simulink library "lib_accessory"  (Simulink 7.9)
settings: Solver=ode45  SolverMode=SingleTasking  StartTime=0.0  StopTime=10.0  RelTol=1e-3
undefined symbols (not defined in the file or in its folder): acc_dcdc_eff, acc_elec_eff, acc_elec_efficiency, acc_elec_pwr, acc_mech_eff, acc_mech_pwr, acc_mech_trq, acc_sindafile, amb_tmp, cyc_mph, ess_on, fc_on, fd_ratio, gb_ratio, load_on, map_spd, max_pwr, pwr_map, tc_gc_to_fc_ratio, time_step, vc_idle_bool, vc_idle_spd, vinf, wh_radius
libraries: lib_accessory x47, lib_cosimulation x29, lib_outputs x11, sub_lib_models x2, simulink3 x2
(part 2 of 3)

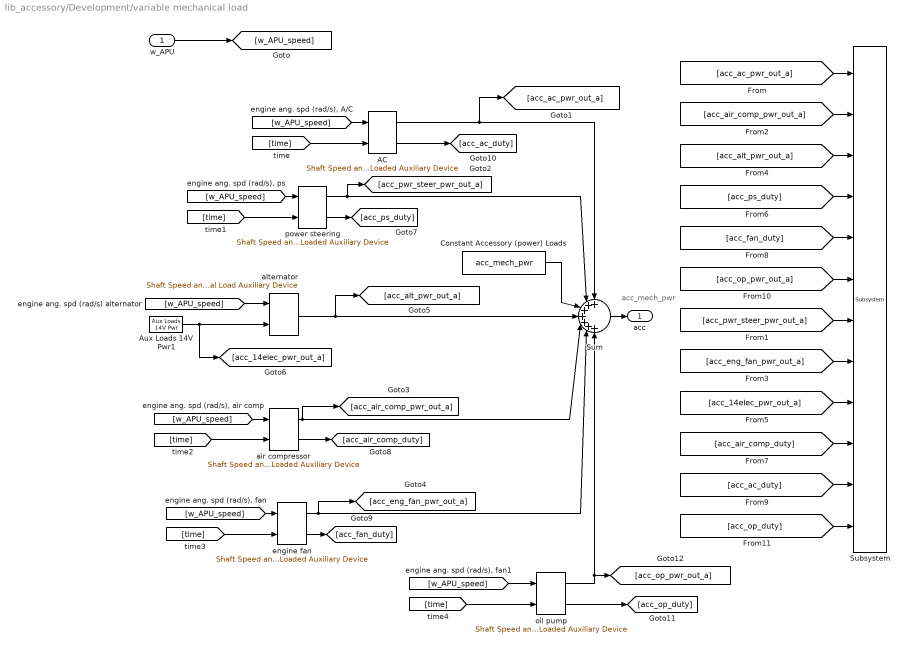
== system lib_accessory/Development/variable mechanical load ==
  note: acc_mech_pwr
  w_APU : Inport
  AC : lib_accessory/SubLibraries/Shaft Speed and Time Loaded Auxiliary Device  acc_duty=acc_ac_dutycycle  pwr_func=acc_ac_pwr_func
  Aux Loads 14V Pwr1 : sub_lib_models/Aux Loads 14V Pwr
      settings: RTWFcnNameOpts=Auto  RTWFileNameOpts=Auto
  Constant Accessory (power) Loads : Constant  Value=acc_mech_pwr
  Subsystem : lib_accessory/SubLibraries/variable accessory load power consumption calculations for conventional mechanical sys. --simulink implementation--/Subsystem
      settings: RTWFcnNameOpts=Auto  RTWFileNameOpts=Auto
  Sum : Sum  Inputs=+++++++  SaturateOnIntegerOverflow=on  InputSameDT=on  OutDataTypeStr=Inherit: Same as first input
  air compressor : lib_accessory/SubLibraries/Shaft Speed and Time Loaded Auxiliary Device  acc_duty=acc_abc_dutycycle  pwr_func=acc_abc_pwr_func
  alternator : lib_accessory/SubLibraries/Shaft Speed and Actual Load Auxiliary Device  conv_eff=acc_acdc_inverter_eff  pwr_func=acc_alt_pwr_func
  engine fan : lib_accessory/SubLibraries/Shaft Speed and Time Loaded Auxiliary Device  acc_duty=acc_ef_dutycycle  pwr_func=acc_ef_pwr_func
  oil pump : lib_accessory/SubLibraries/Shaft Speed and Time Loaded Auxiliary Device  acc_duty=acc_op_dutycycle  pwr_func=acc_op_pwr_func
  power steering : lib_accessory/SubLibraries/Shaft Speed and Time Loaded Auxiliary Device  acc_duty=acc_ps_dutycycle  pwr_func=acc_ps_pwr_func
  acc : Outport
  wires:
  [time] -> AC/2
  [w_APU_speed] -> AC/1
  AC/2 -> [acc_ac_duty]
  AC/1 -> Sum/1, [acc_ac_pwr_out_a]
  Constant Accessory (power) Loads/1 -> Sum/3
  Sum/1 -> acc/1
  [w_APU_speed] -> alternator/1
  air compressor/2 -> [acc_air_comp_duty]
  air compressor/1 -> Sum/5, [acc_air_comp_pwr_out_a]
  [w_APU_speed] -> air compressor/1
  [time] -> air compressor/2
  alternator/1 -> [acc_alt_pwr_out_a], Sum/4
  oil pump/1 -> [acc_op_pwr_out_a], Sum/7
  oil pump/2 -> [acc_op_duty]
  [time] -> oil pump/2
  [w_APU_speed] -> oil pump/1
  engine fan/2 -> [acc_fan_duty]
  [time] -> engine fan/2
  engine fan/1 -> Sum/6, [acc_eng_fan_pwr_out_a]
  [w_APU_speed] -> engine fan/1
  power steering/2 -> [acc_ps_duty]
  [w_APU_speed] -> power steering/1
  [time] -> power steering/2
  power steering/1 -> Sum/2, [acc_pwr_steer_pwr_out_a]
  w_APU/1 -> [w_APU_speed]
  Aux Loads 14V Pwr1/1 -> alternator/2, [acc_14elec_pwr_out_a]
  [acc_ac_pwr_out_a] -> Subsystem/1
  [acc_air_comp_pwr_out_a] -> Subsystem/2
  [acc_alt_pwr_out_a] -> Subsystem/3
  [acc_ps_duty] -> Subsystem/4
  [acc_fan_duty] -> Subsystem/5
  [acc_op_pwr_out_a] -> Subsystem/6
  [acc_pwr_steer_pwr_out_a] -> Subsystem/7
  [acc_eng_fan_pwr_out_a] -> Subsystem/8
  [acc_14elec_pwr_out_a] -> Subsystem/9
  [acc_air_comp_duty] -> Subsystem/10
  [acc_ac_duty] -> Subsystem/11
  [acc_op_duty] -> Subsystem/12

== system lib_accessory/Elec Aux Loads 14V Pwr/BrakeLights ==
  Average Watts : Constant  Value=vinf.AuxLoads.BrakeLights.AverageWatts
  Constant : Constant  Value=0
  Constant1 : Constant
  On : Constant  Value=vinf.AuxLoads.BrakeLights.On
  Product : Product  Inputs=4  SaturateOnIntegerOverflow=on  RndMeth=Zero  InputSameDT=on  OutDataTypeStr=Inherit: Same as first input
  Switch : Switch  SaturateOnIntegerOverflow=on  InputSameDT=on
  Out1 : Outport
  wires:
  Product/1 -> Out1/1
  Constant/1 -> Switch/1
  [F_req] -> Switch/2
  Constant1/1 -> Switch/3
  Average Watts/1 -> Product/4
  [key_on] -> Product/3
  On/1 -> Product/1
  Switch/1 -> Product/2

== system lib_accessory/Elec Aux Loads 14V Pwr/Engine ==
  Average Watts : Constant  Value=vinf.AuxLoads.Engine.AverageWatts
  Memory : Memory
  On : Constant  Value=vinf.AuxLoads.Engine.On
  Product : Product  Inputs=4  SaturateOnIntegerOverflow=on  RndMeth=Zero  InputSameDT=on  OutDataTypeStr=Inherit: Same as first input
  Out1 : Outport
  wires:
  Memory/1 -> Product/2
  [engine_on] -> Memory/1
  [key_on] -> Product/3
  On/1 -> Product/1
  Product/1 -> Out1/1
  Average Watts/1 -> Product/4

== system lib_accessory/Elec Aux Loads 14V Pwr/ExternalLights ==
  Average Watts : Constant  Value=vinf.AuxLoads.ExternalLights.AverageWatts
  On : Constant  Value=vinf.AuxLoads.ExternalLights.On
  Product : Product  Inputs=3  SaturateOnIntegerOverflow=on  RndMeth=Zero  InputSameDT=on  OutDataTypeStr=Inherit: Same as first input
  Subsystem : lib_cosimulation/Subsystem  ModelName='ExternalLights'
  Out1 : Outport
  wires:
  Average Watts/1 -> Product/3
  On/1 -> Product/1
  Subsystem/1 -> Product/2
  Product/1 -> Out1/1

== system lib_accessory/Elec Aux Loads 14V Pwr/FrontHVAC ==
  Average Watts : Constant  Value=vinf.AuxLoads.FrontHVAC.AverageWatts
  On : Constant  Value=vinf.AuxLoads.FrontHVAC.On
  Product : Product  Inputs=3  SaturateOnIntegerOverflow=on  RndMeth=Zero  InputSameDT=on  OutDataTypeStr=Inherit: Same as first input
  Subsystem : lib_cosimulation/Subsystem  ModelName='FrontHVAC'
  Out1 : Outport
  wires:
  Average Watts/1 -> Product/3
  On/1 -> Product/1
  Subsystem/1 -> Product/2
  Product/1 -> Out1/1

== system lib_accessory/Elec Aux Loads 14V Pwr/FrontWipers ==
  Average Watts : Constant  Value=vinf.AuxLoads.FrontWipers.AverageWatts
  On : Constant  Value=vinf.AuxLoads.FrontWipers.On
  Product : Product  Inputs=3  SaturateOnIntegerOverflow=on  RndMeth=Zero  InputSameDT=on  OutDataTypeStr=Inherit: Same as first input
  Subsystem : lib_cosimulation/Subsystem  ModelName='FrontWipers'
  Out1 : Outport
  wires:
  Average Watts/1 -> Product/3
  On/1 -> Product/1
  Subsystem/1 -> Product/2
  Product/1 -> Out1/1

== system lib_accessory/Elec Aux Loads 14V Pwr/HeatedSeats ==
  Average Watts : Constant  Value=vinf.AuxLoads.HeatedSeats.AverageWatts
  Num : Constant  Value=vinf.AuxLoads.HeatedSeats.Num
  On : Constant  Value=vinf.AuxLoads.HeatedSeats.On
  Product : Product  Inputs=4  SaturateOnIntegerOverflow=on  RndMeth=Zero  InputSameDT=on  OutDataTypeStr=Inherit: Same as first input
  Subsystem : lib_cosimulation/Subsystem  ModelName='HeatedSeats'
  Out1 : Outport
  wires:
  Subsystem/1 -> Product/3
  Product/1 -> Out1/1
  Average Watts/1 -> Product/4
  On/1 -> Product/1
  Num/1 -> Product/2

== system lib_accessory/Elec Aux Loads 14V Pwr/Misc ==
  Average Watts : Constant  Value=vinf.AuxLoads.Misc.AverageWatts
  On : Constant  Value=vinf.AuxLoads.Misc.On
  Product : Product  Inputs=3  SaturateOnIntegerOverflow=on  RndMeth=Zero  InputSameDT=on  OutDataTypeStr=Inherit: Same as first input
  Out1 : Outport
  wires:
  Average Watts/1 -> Product/3
  [key_on] -> Product/2
  On/1 -> Product/1
  Product/1 -> Out1/1

== system lib_accessory/Elec Aux Loads 14V Pwr/RadiatorCoolingFan ==
  Average Watts : Constant  Value=vinf.AuxLoads.RadiatorCoolingFan.AverageWatts
  On : Constant  Value=vinf.AuxLoads.RadiatorCoolingFan.On
  Product : Product  Inputs=3  SaturateOnIntegerOverflow=on  RndMeth=Zero  InputSameDT=on  OutDataTypeStr=Inherit: Same as first input
  Subsystem : lib_cosimulation/Subsystem  ModelName='RadiatorCoolingFan'
  Out1 : Outport
  wires:
  Average Watts/1 -> Product/3
  On/1 -> Product/1
  Subsystem/1 -> Product/2
  Product/1 -> Out1/1

== system lib_accessory/Elec Aux Loads 14V Pwr/Radio ==
  Average Watts : Constant  Value=vinf.AuxLoads.Radio.AverageWatts
  Num : Constant  Value=vinf.AuxLoads.Radio.Num
  On : Constant  Value=vinf.AuxLoads.Radio.On
  Product : Product  Inputs=4  SaturateOnIntegerOverflow=on  RndMeth=Zero  InputSameDT=on  OutDataTypeStr=Inherit: Same as first input
  Subsystem : lib_cosimulation/Subsystem  ModelName='Radio'
  Out1 : Outport
  wires:
  Subsystem/1 -> Product/3
  Average Watts/1 -> Product/4
  On/1 -> Product/1
  Num/1 -> Product/2
  Product/1 -> Out1/1

== system lib_accessory/Elec Aux Loads 14V Pwr/RearDefrost ==
  Average Watts : Constant  Value=vinf.AuxLoads.RearDefrost.AverageWatts
  On : Constant  Value=vinf.AuxLoads.RearDefrost.On
  Product : Product  Inputs=3  SaturateOnIntegerOverflow=on  RndMeth=Zero  InputSameDT=on  OutDataTypeStr=Inherit: Same as first input
  Subsystem : lib_cosimulation/Subsystem  ModelName='RearDefrost'
  Out1 : Outport
  wires:
  Subsystem/1 -> Product/2
  Average Watts/1 -> Product/3
  On/1 -> Product/1
  Product/1 -> Out1/1

== system lib_accessory/Elec Aux Loads 14V Pwr/RearHVAC ==
  Average Watts : Constant  Value=vinf.AuxLoads.RearHVAC.AverageWatts
  On : Constant  Value=vinf.AuxLoads.RearHVAC.On
  Product : Product  Inputs=3  SaturateOnIntegerOverflow=on  RndMeth=Zero  InputSameDT=on  OutDataTypeStr=Inherit: Same as first input
  Subsystem : lib_cosimulation/Subsystem  ModelName='RearHVAC'
  Out1 : Outport
  wires:
  Average Watts/1 -> Product/3
  On/1 -> Product/1
  Subsystem/1 -> Product/2
  Product/1 -> Out1/1

== system lib_accessory/Elec Aux Loads 14V Pwr/RearWipers ==
  Average Watts : Constant  Value=vinf.AuxLoads.RearWipers.AverageWatts
  On : Constant  Value=vinf.AuxLoads.RearWipers.On
  Product : Product  Inputs=3  SaturateOnIntegerOverflow=on  RndMeth=Zero  InputSameDT=on  OutDataTypeStr=Inherit: Same as first input
  Subsystem : lib_cosimulation/Subsystem  ModelName='RearWipers'
  Out1 : Outport
  wires:
  Average Watts/1 -> Product/3
  On/1 -> Product/1
  Subsystem/1 -> Product/2
  Product/1 -> Out1/1

== system lib_accessory/Elec Aux Loads 14V Pwr/Starter ==
  Product1 : Product  SaturateOnIntegerOverflow=on  RndMeth=Zero  InputSameDT=on  OutDataTypeStr=Inherit: Same as first input
  Starter : lib_cosimulation/14V Load Control/Starter
      settings: RTWFcnNameOpts=Auto  RTWFileNameOpts=Auto
  starter_load (power) : Constant  Value=vinf.AuxLoads.Starter.AverageWatts
  Out1 : Outport
  wires:
  Starter/1 -> Product1/1
  starter_load (power)/1 -> Product1/2
  Product1/1 -> Out1/1

== system lib_accessory/Elec Aux Loads 14V Pwr/TurnSignals ==
  Average Watts : Constant  Value=vinf.AuxLoads.TurnSignals.AverageWatts
  On : Constant  Value=vinf.AuxLoads.TurnSignals.On
  Product : Product  Inputs=3  SaturateOnIntegerOverflow=on  RndMeth=Zero  InputSameDT=on  OutDataTypeStr=Inherit: Same as first input
  Subsystem : lib_cosimulation/Subsystem  ModelName='TurnSignals'
  Out1 : Outport
  wires:
  Average Watts/1 -> Product/3
  On/1 -> Product/1
  Subsystem/1 -> Product/2
  Product/1 -> Out1/1

== system lib_accessory/Elec Aux Loads HiV Pwr/CurrentLoad1 ==
  Average Watts : Constant  Value=vinf.AuxLoads.CurrentLoad1.AverageWatts
  On : Constant  Value=vinf.AuxLoads.CurrentLoad1.On
  Product : Product  Inputs=3  SaturateOnIntegerOverflow=on  RndMeth=Zero  InputSameDT=on  OutDataTypeStr=Inherit: Same as first input
  Subsystem : lib_cosimulation/Subsystem  ModelName='CurrentLoad1'
  Out1 : Outport
  wires:
  Product/1 -> Out1/1
  Subsystem/1 -> Product/2
  On/1 -> Product/1
  Average Watts/1 -> Product/3

== system lib_accessory/Elec Aux Loads HiV Pwr/PowerLoad1 ==
  Average Watts : Constant  Value=vinf.AuxLoads.PowerLoad1.AverageWatts
  On : Constant  Value=vinf.AuxLoads.PowerLoad1.On
  Product : Product  Inputs=3  SaturateOnIntegerOverflow=on  RndMeth=Zero  InputSameDT=on  OutDataTypeStr=Inherit: Same as first input
  Subsystem : lib_cosimulation/Subsystem  ModelName='PowerLoad1'
  Out1 : Outport
  wires:
  Product/1 -> Out1/1
  On/1 -> Product/1
  Average Watts/1 -> Product/3
  Subsystem/1 -> Product/2

== system lib_accessory/Elec Aux Loads HiV Pwr/PowerLoad2 ==
  Average Watts : Constant  Value=vinf.AuxLoads.PowerLoad2.AverageWatts
  On : Constant  Value=vinf.AuxLoads.PowerLoad2.On
  Product : Product  Inputs=3  SaturateOnIntegerOverflow=on  RndMeth=Zero  InputSameDT=on  OutDataTypeStr=Inherit: Same as first input
  Subsystem : lib_cosimulation/Subsystem  ModelName='PowerLoad2'
  Out1 : Outport
  wires:
  Subsystem/1 -> Product/2
  Average Watts/1 -> Product/3
  On/1 -> Product/1
  Product/1 -> Out1/1

== system lib_accessory/Elec Aux Loads HiV Pwr/PowerLoad3 ==
  Average Watts : Constant  Value=vinf.AuxLoads.PowerLoad3.AverageWatts
  On : Constant  Value=vinf.AuxLoads.PowerLoad3.On
  Product : Product  Inputs=3  SaturateOnIntegerOverflow=on  RndMeth=Zero  InputSameDT=on  OutDataTypeStr=Inherit: Same as first input
  Subsystem : lib_cosimulation/Subsystem  ModelName='PowerLoad3'
  Out1 : Outport
  wires:
  Product/1 -> Out1/1
  On/1 -> Product/1
  Average Watts/1 -> Product/3
  Subsystem/1 -> Product/2

== system lib_accessory/Elec Aux Loads HiV Pwr/SpeedLoad1 ==
  On : Constant  Value=vinf.AuxLoads.SpeedLoad1.On
  Product : Product  Inputs=3  SaturateOnIntegerOverflow=on  RndMeth=Zero  InputSameDT=on  OutDataTypeStr=Inherit: Same as first input
  Subsystem : lib_cosimulation/Subsystem  ModelName='SpeedLoad1'
  "rad/s -> rpm1" : Gain  Gain=60/(2*pi)  SaturateOnIntegerOverflow=on  OutDataTypeStr=Inherit: Same as input  ParamDataTypeStr=Inherit: Same as input
  speed (rpm) vs load (watts) : Lookup  InputValues=[vinf.AuxLoads.SpeedLoad1.Data(1,1),vinf.AuxLoads.SpeedLoad1.Data(2,1)]  Table=[vinf.AuxLoads.SpeedLoad1.Data(1,2),vinf.AuxLoads.SpeedLoad1.Data(2,2)]  SaturateOnIntegerOverflow=on
  Out1 : Outport
  wires:
  Product/1 -> Out1/1
  Subsystem/1 -> Product/2
  On/1 -> Product/1
  speed (rpm) vs load (watts)/1 -> Product/3
  [w_APU_speed] -> "rad/s -> rpm1"/1
  "rad/s -> rpm1"/1 -> speed (rpm) vs load (watts)/1

== system lib_accessory/Elec Aux Loads HiV Pwr/Starter ==
  Product1 : Product  SaturateOnIntegerOverflow=on  RndMeth=Zero  InputSameDT=on  OutDataTypeStr=Inherit: Same as first input
  Starter : Subsystem
  starter_load (power) : Constant  Value=vinf.AuxLoads.Starter.AverageWatts
  Out1 : Outport
  wires:
  Product1/1 -> Out1/1
  starter_load (power)/1 -> Product1/2
  Starter/1(Starter_OnOff_Control) -> Product1/1

== system lib_accessory/Electrical Accessory Loads v2 <acc>/Accessory SDO ==
  data bus : Inport
  Demux : Demux  Outputs=3
  To Workspace : ToWorkspace  VariableName=acc_elec_pwr_r  SampleTime=-1
  To Workspace3 : ToWorkspace  VariableName=acc_elec_pwr_a  SampleTime=-1
  To Workspace4 : ToWorkspace  VariableName=acc_elec_pwr_est  SampleTime=-1
  electrical power logging : lib_accessory/SubLibraries/electrical power logging  eff=acc_mech_eff
  wires:
  data bus/1 -> Demux/1
  Demux/1 -> To Workspace/1
  Demux/2 -> To Workspace3/1, electrical power logging/1
  Demux/3 -> To Workspace4/1

== system lib_accessory/Electrical Accessory Loads v2 <acc>/Block NOTES ==
  note: In terms of an interface, the model assumes electrical power generated from
      | a powersource (or powersources)
      |
      | This model takes in requested driveline electrical power output requests and
      | augments power to account for electrically driven accessories.
      |
      | The power passed along down to the driveline is only power to move the
      | vehicle.
  note: This is the electrical auxiliary loads model.

== system lib_accessory/Electrical Accessory Loads v2 <acc>/backward model ==
  note: Pwr, W, powersource out
  note: P, W, for driveline
  note: Power Electrical
      | Accessory
      | (W)
  pwr_in : Inport
  on/off : Inport  Port=2
  Constant : Constant  Value=load_on
  Product : Product  Inputs=***  SaturateOnIntegerOverflow=on  RndMeth=Zero  InputSameDT=on  OutDataTypeStr=Inherit: Same as first input
  Sum : Sum  Inputs=|++  SaturateOnIntegerOverflow=on  InputSameDT=on  OutDataTypeStr=Inherit: Same as first input
  electrical accessories (W) : Subsystem  BlockChoice=Electrical Accessories: Time Variable
      settings: AttributesFormatString=%<BlockChoice>  TemplateBlock=lib_accessory/electrical accessories (W)  MemberBlocks=Electrical Accessories: Constant,Electrical Accessories: Time Variable
      mask Display: image(imread('bdi_acc_elec.bmp'))
  elec_out : Outport
  elec_acc_out : Outport  Port=2
  wires:
  Sum/1 -> elec_out/1
  pwr_in/1 -> Sum/1
  electrical accessories (W)/1(P_elec_acc) -> Product/1
  on/off/1 -> Product/2
  Constant/1 -> Product/3
  Product/1 -> elec_acc_out/1, Sum/2

== system lib_accessory/Electrical Accessory Loads v2 <acc>/forward model ==
  note: Power to driveline
  note: Power Available
  note: electric
      | accessory
      | power (W)
  note: This calculation assumes that the power provider is never so power limited as to
      | not be able to provide at least the value of acc_pwr_in.
  note: ASSUMPTIONS
  pwr_in : Inport
  acc_pwr_in : Inport  Port=2
  Sum : Sum  Inputs=|+-  SaturateOnIntegerOverflow=on  InputSameDT=on  OutDataTypeStr=Inherit: Same as first input
  pwr_out : Outport
  acc_pwr_out : Outport  Port=2
  wires:
  Sum/1 -> pwr_out/1
  pwr_in/1 -> Sum/1
  acc_pwr_in/1 -> Sum/2, acc_pwr_out/1

== system lib_accessory/Mechanical Accessory Loads v2 <acc>/Accessory SDO ==
  data bus : Inport
  Demux : Demux  Outputs=6
  To Workspace : ToWorkspace  VariableName=acc_mech_trq_r  SampleTime=-1
  To Workspace1 : ToWorkspace  VariableName=acc_mech_pwr_a  SampleTime=-1
  To Workspace2 : ToWorkspace  VariableName=acc_mech_trq_est  SampleTime=-1
  To Workspace3 : ToWorkspace  VariableName=acc_mech_pwr_r  SampleTime=-1
  To Workspace4 : ToWorkspace  VariableName=acc_mech_trq_a  SampleTime=-1
  To Workspace5 : ToWorkspace  VariableName=acc_mech_pwr_est  SampleTime=-1
  mechanical power logging : lib_accessory/SubLibraries/mechanical power logging  eff=acc_mech_eff
  wires:
  data bus/1 -> Demux/1
  Demux/4 -> mechanical power logging/1, To Workspace1/1
  Demux/1 -> To Workspace/1
  Demux/2 -> To Workspace3/1
  Demux/3 -> To Workspace4/1
  Demux/5 -> To Workspace2/1
  Demux/6 -> To Workspace5/1

== system lib_accessory/Mechanical Accessory Loads v2 <acc>/Block NOTES ==
  note: This is the mechanical auxiliary loads model.
  note: In terms of an interface, the model assumes belt-driven mechanical loads
      | that run off of a prime mover shaft (e.g., engine shaft)
      |
      | This model takes in requested driveline torque and speed requests and
      | augments torque due to belt driven accessories.
      |
      | The torque passed along down to the driveline is only torque to move the
      | vehicle.
  note: A third input is given for accessory load speed. This is done so that
      | the accessory block can use fc_spd_est which is an estimated vehicle speed
      | (equal to fc_spd_out under normal circumstances).
      | Using fc_spd_est provides total compatibility with ADVISOR v3.2
  note: In this model, only one speed is used to predict accessory
      | loading. The forward model is "dummied" out.

== system lib_accessory/Mechanical Accessory Loads v2 <acc>/backward model ==
  note: w_apu, rad/s
  note: T, Nm, accessory
  note: T, Nm, driveline
  note: T, Nm, shaft out
  note: Power, W, input to accessory
  trq_in : Inport
  spd_in : Inport  Port=2
  acc on/off : Inport  Port=3
  Product : Product  Inputs=**  SaturateOnIntegerOverflow=on  RndMeth=Zero  InputSameDT=on  OutDataTypeStr=Inherit: Same as first input
  Product1 : Product  Inputs=**  SaturateOnIntegerOverflow=on  RndMeth=Zero  InputSameDT=on  OutDataTypeStr=Inherit: Same as first input
  Sum : Sum  Inputs=|++  SaturateOnIntegerOverflow=on  InputSameDT=on  OutDataTypeStr=Inherit: Same as first input
  acc_mech_var_loads : ToWorkspace  VariableName=acc_mech_var_load  SampleTime=-1  SaveFormat=Structure
  mechanical accessories (Nm) : Subsystem  BlockChoice=Mechanical Accessories: Speed Dependant and Variable Electrical
      settings: AttributesFormatString=%<BlockChoice>  TemplateBlock=lib_accessory/mechanical accessories (Nm)  MemberBlocks=Mechanical Accessories: Const Mech Var Elect,Mechanical Accessories: Constant Mechanical & Electrical,Mechanical Accessories: Speed Dependant and Variable Electrical,Saber Dual Voltage Cosim,Saber Single Voltage Cosim,SindaTransAC
      mask Display: image(imread('bdi_acc_pic_cs.bmp'))
  trq_out : Outport
  acc_mech_trq_r : Outport  Port=2
  acc_mech_pwr_r : Outport  Port=3
  wires:
  spd_in/1 -> mechanical accessories (Nm)/1(w_APU)
  trq_in/1 -> Sum/1
  Sum/1 -> trq_out/1
  Product/1 -> acc_mech_trq_r/1, Sum/2
  mechanical accessories (Nm)/1(T_acc) -> Product/2
  Product1/1 -> acc_mech_pwr_r/1
  mechanical accessories (Nm)/2(P_mech_acc) -> Product1/1
  acc on/off/1 -> [acc_on]
  [acc_on] -> Product/1
  [acc_on] -> Product1/2
  mechanical accessories (Nm)/3(probes) -> acc_mech_var_loads/1

== system lib_accessory/Mechanical Accessory Loads v2 <acc>/forward model ==
  note: acc speed, rad/s
  note: T, Nm, accessory
  note: driveline and
      | acc torque, Nm
  note: T, Nm, shaft out
  note: Power, W, input to accessory
  note: This simplistic model may not correctly account for accessory torque and/or power
      | when the upstream torque provider is torque or speed limited
  note: NOTES
  note: acc torque, Nm
  trq_in : Inport
  spd_in : Inport  Port=2
  acc_trq_req : Inport  Port=3
  Product1 : Product  Inputs=**  SaturateOnIntegerOverflow=on  RndMeth=Zero  InputSameDT=on  OutDataTypeStr=Inherit: Same as first input
  Sum : Sum  Inputs=|+-  SaturateOnIntegerOverflow=on  InputSameDT=on  OutDataTypeStr=Inherit: Same as first input
  trq_out : Outport
  acc_mech_trq_a : Outport  Port=2
  acc_mech_pwr_a : Outport  Port=3
  wires:
  spd_in/1 -> [acc_spd]
  Sum/1 -> trq_out/1
  Product1/1 -> acc_mech_pwr_a/1
  [acc_trq_r] -> acc_mech_trq_a/1, Sum/2, Product1/1
  [acc_spd] -> Product1/2
  trq_in/1 -> [pm_trq_a]
  acc_trq_req/1 -> [acc_trq_r]
  [pm_trq_a] -> Sum/1

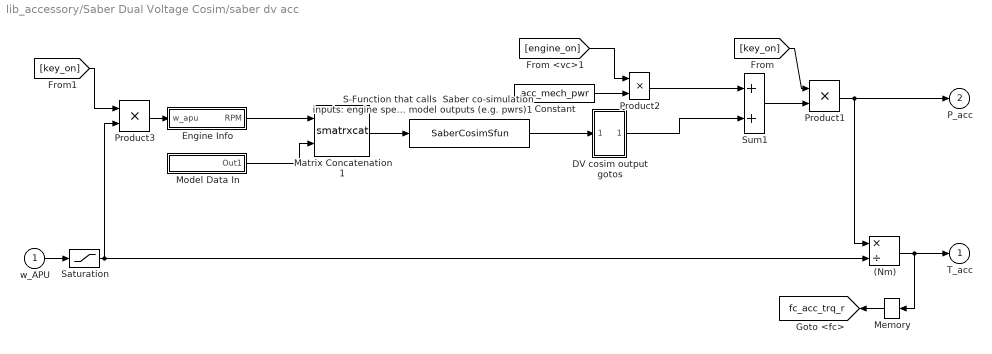
== system lib_accessory/Saber Dual Voltage Cosim/saber dv acc ==
  w_APU : Inport
  (Nm) : Product  Inputs=*/  SaturateOnIntegerOverflow=on  RndMeth=Zero  InputSameDT=on  OutDataTypeStr=Inherit: Same as first input
  Constant : Constant  Value=acc_mech_pwr
  DV cosim output gotos : Subsystem
  Engine Info : Subsystem
  Matrix Concatenation1 : S-Function  FunctionName=smatrxcat  Parameters=numInports,catMethod  EnableBusSupport=off  mask(Matrix Concatenation){numInports=2, catMethod=Horizontal}
      mask prompts: numInports "Number of inputs:"; catMethod "Concatenation method:"
      mask help: Perform horizontal or vertical concatenation. 1-D vector input signals are treated as column vectors, i.e., [Mx1] matrices. The output is always a matrix.
      mask init:
      | xy = matrxcatmask('icon');
      mask StyleString: edit,popup(Horizontal|Vertical)
      mask Display:
      | plot(xy.x,xy.y);
      | text(0.15,0.86,xy.label);
  Memory : Memory
  Model Data In : Subsystem
      mask Display: disp('14V/42V acc')
  Product1 : Product  SaturateOnIntegerOverflow=on  RndMeth=Zero  InputSameDT=on  OutDataTypeStr=Inherit: Same as first input
  Product2 : Product  SaturateOnIntegerOverflow=on  RndMeth=Zero  InputSameDT=on  OutDataTypeStr=Inherit: Same as first input
  Product3 : Product  SaturateOnIntegerOverflow=on  RndMeth=Zero  InputSameDT=on  OutDataTypeStr=Inherit: Same as first input
  S-Function that calls  Saber co-simulation inputs: engine speed (rad/s) load parameters outputs: accessory power model outputs (e.g. pwrs)1 : S-Function  FunctionName=SaberCosimSfun  Parameters=vinf.tmppath,time_step,'SaberCosimIO_DV'  EnableBusSupport=off
  Saturation : Saturate  UpperLimit=inf  LowerLimit=0
  Sum1 : Sum  SaturateOnIntegerOverflow=on  InputSameDT=on  OutDataTypeStr=Inherit: Same as first input
  T_acc : Outport  InitialOutput=0
  P_acc : Outport  Port=2  InitialOutput=0
  tag scope: fc_acc_trq_r=global
  wires:
  Product3/1 -> Engine Info/1(w_apu)
  [key_on] -> Product3/1
  DV cosim output gotos/1(Out1) -> Sum1/2
  Product1/1 -> (Nm)/1, P_acc/1
  [key_on] -> Product1/1
  Sum1/1 -> Product1/2
  Product2/1 -> Sum1/1
  [engine_on] -> Product2/1
  Constant/1 -> Product2/2
  (Nm)/1 -> T_acc/1, Memory/1
  Memory/1 -> [fc_acc_trq_r]
  w_APU/1 -> Saturation/1
  Saturation/1 -> Product3/2, (Nm)/2
  S-Function that calls  Saber co-simulation inputs: engine speed (rad/s) load parameters outputs: accessory power model outputs (e.g. pwrs)1/1 -> DV cosim output gotos/1(In1)
  Matrix Concatenation1/1 -> S-Function that calls  Saber co-simulation inputs: engine speed (rad/s) load parameters outputs: accessory power model outputs (e.g. pwrs)1/1
  Engine Info/1(RPM) -> Matrix Concatenation1/1
  Model Data In/1(Out1) -> Matrix Concatenation1/2

== system lib_accessory/Saber Single Voltage Cosim/saber sv acc ==
  w_APU : Inport
  (Nm) : Product  Inputs=*/  SaturateOnIntegerOverflow=on  RndMeth=Zero  InputSameDT=on  OutDataTypeStr=Inherit: Same as first input
  Constant : Constant  Value=acc_mech_pwr
  Engine Info : Subsystem
  Matrix Concatenation1 : S-Function  FunctionName=smatrxcat  Parameters=numInports,catMethod  EnableBusSupport=off  mask(Matrix Concatenation){numInports=2, catMethod=Horizontal}
      mask prompts: numInports "Number of inputs:"; catMethod "Concatenation method:"
      mask help: Perform horizontal or vertical concatenation. 1-D vector input signals are treated as column vectors, i.e., [Mx1] matrices. The output is always a matrix.
      mask init:
      | xy = matrxcatmask('icon');
      mask StyleString: edit,popup(Horizontal|Vertical)
      mask Display:
      | plot(xy.x,xy.y);
      | text(0.15,0.86,xy.label);
  Memory : Memory
  Product1 : Product  SaturateOnIntegerOverflow=on  RndMeth=Zero  InputSameDT=on  OutDataTypeStr=Inherit: Same as first input
  Product2 : Product  SaturateOnIntegerOverflow=on  RndMeth=Zero  InputSameDT=on  OutDataTypeStr=Inherit: Same as first input
  Product3 : Product  SaturateOnIntegerOverflow=on  RndMeth=Zero  InputSameDT=on  OutDataTypeStr=Inherit: Same as first input
  S-Function that calls  Saber co-simulation inputs: engine speed (rad/s) load parameters outputs: accessory power model outputs (e.g. pwrs) : S-Function  FunctionName=SaberCosimSfun  Parameters=vinf.tmppath,time_step,'SaberCosimIO_SV'  EnableBusSupport=off
  SV Model Data In : Subsystem
      mask Display: disp('14V acc')
  SV cosim output gotos : Subsystem
  Saturation : Saturate  UpperLimit=inf  LowerLimit=0
  Sum1 : Sum  SaturateOnIntegerOverflow=on  InputSameDT=on  OutDataTypeStr=Inherit: Same as first input
  T_acc : Outport  InitialOutput=0
  P_acc : Outport  Port=2  InitialOutput=0
  tag scope: fc_acc_trq_r=global
  wires:
  Product3/1 -> Engine Info/1(w_apu)
  [key_on] -> Product3/1
  SV cosim output gotos/1(Out1) -> Sum1/2
  SV Model Data In/1(Out1) -> Matrix Concatenation1/2
  Engine Info/1(RPM) -> Matrix Concatenation1/1
  Matrix Concatenation1/1 -> S-Function that calls  Saber co-simulation inputs: engine speed (rad/s) load parameters outputs: accessory power model outputs (e.g. pwrs)/1
  S-Function that calls  Saber co-simulation inputs: engine speed (rad/s) load parameters outputs: accessory power model outputs (e.g. pwrs)/1 -> SV cosim output gotos/1(In1)
  Saturation/1 -> Product3/2, (Nm)/2
  w_APU/1 -> Saturation/1
  Memory/1 -> [fc_acc_trq_r]
  (Nm)/1 -> Memory/1, T_acc/1
  Constant/1 -> Product2/2
  [engine_on] -> Product2/1
  Product2/1 -> Sum1/1
  Sum1/1 -> Product1/2
  [key_on] -> Product1/1
  Product1/1 -> P_acc/1, (Nm)/1

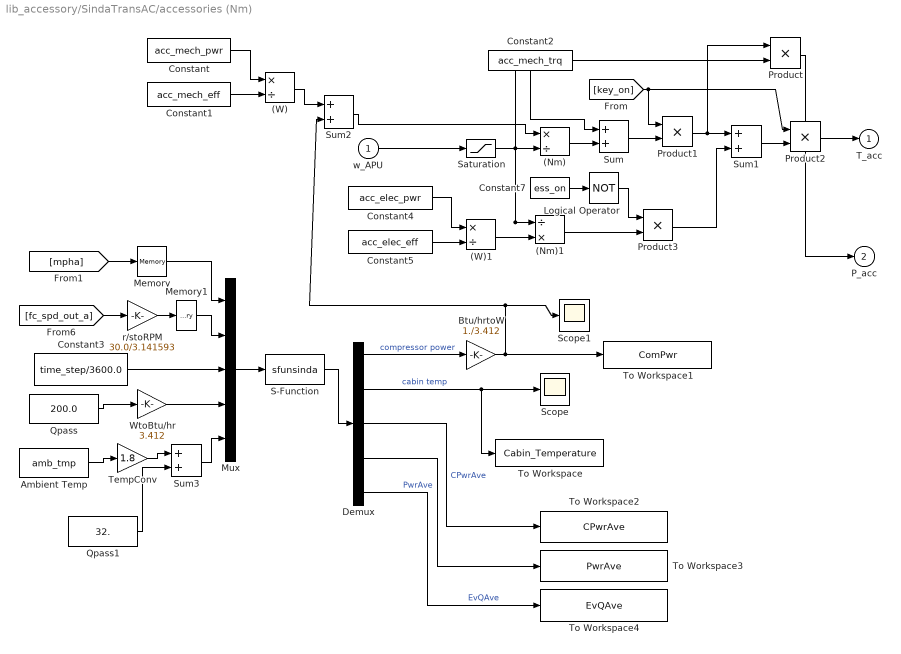
== system lib_accessory/SindaTransAC/accessories (Nm) ==
  w_APU : Inport
  (Nm) : Product  Inputs=*/  SaturateOnIntegerOverflow=on  RndMeth=Zero  InputSameDT=on  OutDataTypeStr=Inherit: Same as first input
  (Nm)1 : Product  Inputs=/*  SaturateOnIntegerOverflow=on  RndMeth=Zero  InputSameDT=on  OutDataTypeStr=Inherit: Same as first input
  (W) : Product  Inputs=*/  SaturateOnIntegerOverflow=on  RndMeth=Zero  InputSameDT=on  OutDataTypeStr=Inherit: Same as first input
  (W)1 : Product  Inputs=*/  SaturateOnIntegerOverflow=on  RndMeth=Zero  InputSameDT=on  OutDataTypeStr=Inherit: Same as first input
  Ambient Temp : Constant  Value=amb_tmp
  Btu/hrtoW : Gain  Gain=1./3.412  SaturateOnIntegerOverflow=on  OutDataTypeStr=Inherit: Same as input  ParamDataTypeStr=Inherit: Same as input
  Constant : Constant  Value=acc_mech_pwr
  Constant1 : Constant  Value=acc_mech_eff
  Constant2 : Constant  Value=acc_mech_trq
  Constant3 : Constant  Value=time_step/3600.0
  Constant4 : Constant  Value=acc_elec_pwr
  Constant5 : Constant  Value=acc_elec_eff
  Constant7 : Constant  Value=ess_on
  Demux : Demux  Outputs=5
  Logical Operator : Logic  Operator=NOT
  Memory : Memory  X0=45.0
  Memory1 : Memory  X0=600.
  Mux : Mux  Inputs=5
  Product{,1..3} (4 alike) : Product  SaturateOnIntegerOverflow=on  RndMeth=Zero  InputSameDT=on  OutDataTypeStr=Inherit: Same as first input
  Qpass : Constant  Value=200.0
  Qpass1 : Constant  Value=32.
  S-Function : S-Function  FunctionName=sfunsinda  Parameters=sindafile  EnableBusSupport=off
  Saturation : Saturate  UpperLimit=inf  LowerLimit=vc_idle_spd+eps
  Scope : Scope
      settings: YMin=130  YMax=170
  Scope1 : Scope
  Sum{,1..3} (4 alike) : Sum  SaturateOnIntegerOverflow=on  InputSameDT=on  OutDataTypeStr=Inherit: Same as first input
  TempConv : Gain  Gain=1.8  SaturateOnIntegerOverflow=on  OutDataTypeStr=Inherit: Same as input  ParamDataTypeStr=Inherit: Same as input
  To Workspace : ToWorkspace  VariableName=Cabin_Temperature  SampleTime=-1
  To Workspace1 : ToWorkspace  VariableName=ComPwr  SampleTime=-1
  To Workspace2 : ToWorkspace  VariableName=CPwrAve  SampleTime=-1
  To Workspace3 : ToWorkspace  VariableName=PwrAve  SampleTime=-1
  To Workspace4 : ToWorkspace  VariableName=EvQAve  SampleTime=-1
  WtoBtu/hr : Gain  Gain=3.412  SaturateOnIntegerOverflow=on  OutDataTypeStr=Inherit: Same as input  ParamDataTypeStr=Inherit: Same as input
  r/stoRPM : Gain  Gain=30.0/3.141593  SaturateOnIntegerOverflow=on  OutDataTypeStr=Inherit: Same as input  ParamDataTypeStr=Inherit: Same as input
  T_acc : Outport  InitialOutput=0
  P_acc : Outport  Port=2  InitialOutput=0
  wires:
  Mux/1 -> S-Function/1
  S-Function/1 -> Demux/1
  [fc_spd_out_a] -> r/stoRPM/1
  Qpass/1 -> WtoBtu/hr/1
  WtoBtu/hr/1 -> Mux/4
  Product1/1 -> Product/1, Sum1/1
  Sum1/1 -> Product2/2
  Logical Operator/1 -> Product3/1
  Product3/1 -> Sum1/2
  Product/1 -> P_acc/1
  (Nm)1/1 -> Product3/2
  Constant7/1 -> Logical Operator/1
  (W)1/1 -> (Nm)1/2
  Constant4/1 -> (W)1/1
  Constant5/1 -> (W)1/2
  Product2/1 -> T_acc/1
  [key_on] -> Product2/1, Product1/1
  Sum/1 -> Product1/2
  (Nm)/1 -> Sum/2
  Saturation/1 -> Product/2, (Nm)1/1, (Nm)/2
  w_APU/1 -> Saturation/1
  Constant2/1 -> Sum/1
  (W)/1 -> Sum2/1
  Sum2/1 -> (Nm)/1
  Constant/1 -> (W)/1
  Constant1/1 -> (W)/2
  Demux/2 -> To Workspace/1, Scope/1  "cabin temp"
  Ambient Temp/1 -> TempConv/1
  TempConv/1 -> Sum3/1
  Qpass1/1 -> Sum3/2
  Sum3/1 -> Mux/5
  Demux/1 -> Btu/hrtoW/1  "compressor power"
  [mpha] -> Memory/1
  Memory/1 -> Mux/1
  r/stoRPM/1 -> Memory1/1
  Memory1/1 -> Mux/2
  Constant3/1 -> Mux/3
  Btu/hrtoW/1 -> Sum2/2, Scope1/1, To Workspace1/1
  Demux/3 -> To Workspace2/1  "CPwrAve"
  Demux/4 -> To Workspace3/1  "PwrAve"
  Demux/5 -> To Workspace4/1  "EvQAve"

== system lib_accessory/SubLibraries/Shaft Speed and Actual Load Auxiliary Device ==
  angular  speed of engine  shaft (rad/s) : Inport
  load on device (W) : Inport  Port=2
  Gain : Gain  Gain=1/conv_eff  SaturateOnIntegerOverflow=on  OutDataTypeStr=Inherit: Same as input  ParamDataTypeStr=Inherit: Same as input
  Mux : Mux  Inputs=2
  device power requirements : MATLABFcn  MATLABFcn=feval(pwr_func, u(1), u(2))  OutputDimensions=1  OutputSignalType=real
  powr required by device (W) : Outport
  wires:
  angular  speed of engine  shaft (rad/s)/1 -> Mux/1
  Gain/1 -> Mux/2
  load on device (W)/1 -> Gain/1
  device power requirements/1 -> powr required by device (W)/1
  Mux/1 -> device power requirements/1

== system lib_accessory/SubLibraries/Shaft Speed and Actual Load Auxiliary Device--lookuptable ==
  angular  speed of engine  shaft (rad/s) : Inport
  load on device (W) : Inport  Port=2
  Constant : Constant  Value=0.0
  Constant1 : Constant  Value=eps
  Gain : Gain  Gain=1/conv_eff  SaturateOnIntegerOverflow=on  OutDataTypeStr=Inherit: Same as input  ParamDataTypeStr=Inherit: Same as input
  Look-Up Table : Lookup  InputValues=map_spd  Table=max_pwr  SaturateOnIntegerOverflow=on
  Look-Up Table (2-D) : simulink3/Functions & Tables/Look-Up Table (2-D)  x=map_spd  y=map_load  t=pwr_map
  Product : Product  Inputs=*/  SaturateOnIntegerOverflow=on  RndMeth=Zero  InputSameDT=on  OutDataTypeStr=Inherit: Same as first input
  Relational Operator : RelationalOperator  Operator=~=  InputSameDT=on
  Saturation : Saturate  UpperLimit=1.0  LowerLimit=0.0
  Saturation1 : Saturate  UpperLimit=maxSpd  LowerLimit=minSpd
  Switch : Switch  Threshold=0.5  SaturateOnIntegerOverflow=on  InputSameDT=on
  powr required by device (W) : Outport
  wires:
  load on device (W)/1 -> Gain/1
  Look-Up Table (2-D)/1 -> powr required by device (W)/1
  angular  speed of engine  shaft (rad/s)/1 -> Saturation1/1
  [spd] -> Look-Up Table (2-D)/1
  Saturation1/1 -> [spd]
  Gain/1 -> Product/1
  [spd] -> Look-Up Table/1
  Product/1 -> Saturation/1
  Saturation/1 -> Look-Up Table (2-D)/2
  Look-Up Table/1 -> Relational Operator/1, Switch/1
  Constant/1 -> Relational Operator/2
  Relational Operator/1 -> Switch/2
  Constant1/1 -> Switch/3
  Switch/1 -> Product/2

== system lib_accessory/SubLibraries/Shaft Speed and Time Loaded Auxiliary Device ==
  angular  speed of engine  shaft (rad/s) : Inport
  elapsed time since start of simulation (s) : Inport  Port=2
  Mux : Mux  Inputs=2
  Sat : Saturate  UpperLimit=1.0  LowerLimit=0.0
  device duty  schedule by time : Subsystem  mask(Repeating table){t=acc_duty(:,1), y=acc_duty(:,2)}
      mask prompts: t "Input values:"; y "Output values:"
      mask help:
      | Repeating table.
      | Enter values of input and output for first cycle.
      mask init:
      | period = max(@1);
      mask Help: Repeats cycle given in table. Input values should be monotonically increasing.
  device power requirements : MATLABFcn  MATLABFcn=feval(pwr_func, u(1), u(2))  OutputDimensions=1  OutputSignalType=real
  powr required by device (W) : Outport
  "duty cycle (1=\"on full power\" & 0=\"off\")" : Outport  Port=2
  wires:
  Mux/1 -> device power requirements/1
  angular  speed of engine  shaft (rad/s)/1 -> Mux/1
  device power requirements/1 -> powr required by device (W)/1
  elapsed time since start of simulation (s)/1 -> device duty  schedule by time/1(distance travelled (m))
  device duty  schedule by time/1(out_1) -> Sat/1
  Sat/1 -> Mux/2, "duty cycle (1=\"on full power\" & 0=\"off\")"/1

== system lib_accessory/SubLibraries/Shaft Speed and Time Loaded Auxiliary Device--lookuptable ==
  angular  speed of engine  shaft (rad/s) : Inport
  elapsed time since start of simulation (s) : Inport  Port=2
  Look-Up Table (2-D) : Lookup2D  RowIndex=map_spd  ColumnIndex=map_load  Table=pwr_map  SaturateOnIntegerOverflow=on  InputSameDT=on
  Sat : Saturate  UpperLimit=1.0  LowerLimit=0.0
  Sat1 : Saturate  UpperLimit=maxSpd  LowerLimit=minSpd
  device duty  schedule by time : Subsystem  mask(Repeating table){t=acc_duty(:,1), y=acc_duty(:,2)}
      mask prompts: t "Input values:"; y "Output values:"
      mask help:
      | Repeating table.
      | Enter values of input and output for first cycle.
      mask init:
      | period = max(t);
      mask Help: Repeats cycle given in table. Input values should be monotonically increasing.
  powr required by device (W) : Outport
  "duty cycle (1=\"on full power\" & 0=\"off\")" : Outport  Port=2
  wires:
  Look-Up Table (2-D)/1 -> powr required by device (W)/1
  elapsed time since start of simulation (s)/1 -> device duty  schedule by time/1(distance travelled (m))
  device duty  schedule by time/1(out_1) -> Sat/1
  Sat/1 -> "duty cycle (1=\"on full power\" & 0=\"off\")"/1, Look-Up Table (2-D)/2
  angular  speed of engine  shaft (rad/s)/1 -> Sat1/1
  Sat1/1 -> Look-Up Table (2-D)/1

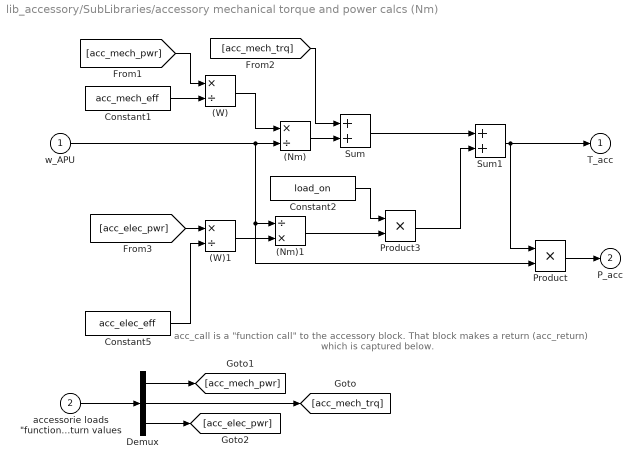
== system lib_accessory/SubLibraries/accessory mechanical torque and power calcs (Nm) ==
  note: acc_call is a "function call" to the
      | accessory block. That block makes
      | a return (acc_return) which is captured below.
  w_APU : Inport
  "accessorie loads \"function\" return values" : Inport  Port=2
  (Nm) : Product  Inputs=*/  SaturateOnIntegerOverflow=on  RndMeth=Zero  InputSameDT=on  OutDataTypeStr=Inherit: Same as first input
  (Nm)1 : Product  Inputs=/*  SaturateOnIntegerOverflow=on  RndMeth=Zero  InputSameDT=on  OutDataTypeStr=Inherit: Same as first input
  (W) : Product  Inputs=*/  SaturateOnIntegerOverflow=on  RndMeth=Zero  InputSameDT=on  OutDataTypeStr=Inherit: Same as first input
  (W)1 : Product  Inputs=*/  SaturateOnIntegerOverflow=on  RndMeth=Zero  InputSameDT=on  OutDataTypeStr=Inherit: Same as first input
  Constant1 : Constant  Value=acc_mech_eff
  Constant2 : Constant  Value=load_on
  Constant5 : Constant  Value=acc_elec_eff
  Demux : Demux  Outputs=3
  Product : Product  SaturateOnIntegerOverflow=on  RndMeth=Zero  InputSameDT=on  OutDataTypeStr=Inherit: Same as first input
  Product3 : Product  SaturateOnIntegerOverflow=on  RndMeth=Zero  InputSameDT=on  OutDataTypeStr=Inherit: Same as first input
  Sum : Sum  SaturateOnIntegerOverflow=on  InputSameDT=on  OutDataTypeStr=Inherit: Same as first input
  Sum1 : Sum  SaturateOnIntegerOverflow=on  InputSameDT=on  OutDataTypeStr=Inherit: Same as first input
  T_acc : Outport  InitialOutput=0
  P_acc : Outport  Port=2  InitialOutput=0
  wires:
  "accessorie loads \"function\" return values"/1 -> Demux/1
  Demux/3 -> [acc_elec_pwr]
  Demux/1 -> [acc_mech_pwr]
  Demux/2 -> [acc_mech_trq]
  Product/1 -> P_acc/1
  (W)/1 -> (Nm)/1
  Constant1/1 -> (W)/2
  [acc_mech_pwr] -> (W)/1
  (Nm)/1 -> Sum/2
  Sum/1 -> Sum1/1
  Sum1/1 -> Product/1, T_acc/1
  Constant5/1 -> (W)1/2
  (W)1/1 -> (Nm)1/2
  (Nm)1/1 -> Product3/2
  Product3/1 -> Sum1/2
  Constant2/1 -> Product3/1
  [acc_mech_trq] -> Sum/1
  w_APU/1 -> (Nm)1/1, Product/2, (Nm)/2
  [acc_elec_pwr] -> (W)1/1

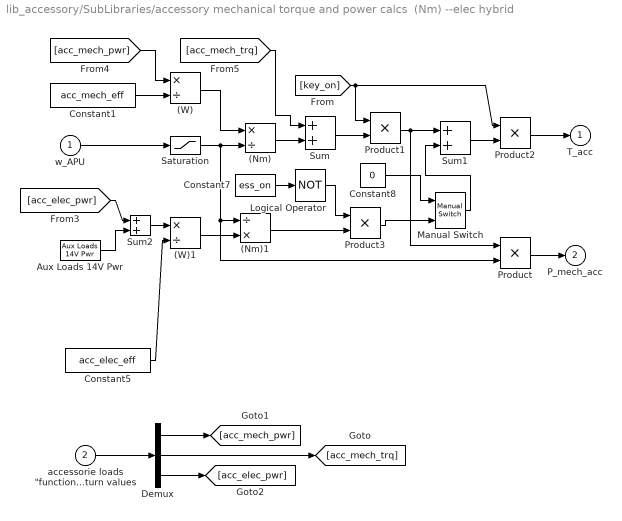
== system lib_accessory/SubLibraries/accessory mechanical torque and power calcs  (Nm) --elec hybrid ==
  w_APU : Inport
  "accessorie loads \"function\" return values" : Inport  Port=2
  (Nm) : Product  Inputs=*/  SaturateOnIntegerOverflow=on  RndMeth=Zero  InputSameDT=on  OutDataTypeStr=Inherit: Same as first input
  (Nm)1 : Product  Inputs=/*  SaturateOnIntegerOverflow=on  RndMeth=Zero  InputSameDT=on  OutDataTypeStr=Inherit: Same as first input
  (W) : Product  Inputs=*/  SaturateOnIntegerOverflow=on  RndMeth=Zero  InputSameDT=on  OutDataTypeStr=Inherit: Same as first input
  (W)1 : Product  Inputs=*/  SaturateOnIntegerOverflow=on  RndMeth=Zero  InputSameDT=on  OutDataTypeStr=Inherit: Same as first input
  Aux Loads 14V Pwr : sub_lib_models/Aux Loads 14V Pwr
      settings: RTWFcnNameOpts=Auto  RTWFileNameOpts=Auto
  Constant1 : Constant  Value=acc_mech_eff
  Constant5 : Constant  Value=acc_elec_eff
  Constant7 : Constant  Value=ess_on
  Constant8 : Constant  Value=0
  Demux : Demux  Outputs=3
  Logical Operator : Logic  Operator=NOT
  Manual Switch : simulink3/Nonlinear/Manual Switch  sw=1  action=0
  Product{,1..3} (4 alike) : Product  SaturateOnIntegerOverflow=on  RndMeth=Zero  InputSameDT=on  OutDataTypeStr=Inherit: Same as first input
  Saturation : Saturate  UpperLimit=inf  LowerLimit=vc_idle_spd+eps
  Sum : Sum  SaturateOnIntegerOverflow=on  InputSameDT=on  OutDataTypeStr=Inherit: Same as first input
  Sum1 : Sum  SaturateOnIntegerOverflow=on  InputSameDT=on  OutDataTypeStr=Inherit: Same as first input
  Sum2 : Sum  SaturateOnIntegerOverflow=on  InputSameDT=on  OutDataTypeStr=Inherit: Same as first input
  T_acc : Outport  InitialOutput=0
  P_mech_acc : Outport  Port=2  InitialOutput=0
  wires:
  Logical Operator/1 -> Product3/1
  (Nm)1/1 -> Product3/2
  Constant7/1 -> Logical Operator/1
  (W)1/1 -> (Nm)1/2
  Constant5/1 -> (W)1/2
  Product2/1 -> T_acc/1
  [key_on] -> Product2/1, Product1/1
  Sum1/1 -> Product2/2
  Sum/1 -> Product1/2
  (Nm)/1 -> Sum/2
  Saturation/1 -> (Nm)/2, Product/2, (Nm)1/1
  w_APU/1 -> Saturation/1
  [acc_mech_pwr] -> (W)/1
  Constant1/1 -> (W)/2
  (W)/1 -> (Nm)/1
  [acc_mech_trq] -> Sum/1
  Product/1 -> P_mech_acc/1
  Product1/1 -> Product/1, Sum1/1
  Product3/1 -> Manual Switch/2
  Manual Switch/1 -> Sum1/2
  Constant8/1 -> Manual Switch/1
  Sum2/1 -> (W)1/1
  [acc_elec_pwr] -> Sum2/1
  Aux Loads 14V Pwr/1 -> Sum2/2
  "accessorie loads \"function\" return values"/1 -> Demux/1
  Demux/3 -> [acc_elec_pwr]
  Demux/1 -> [acc_mech_pwr]
  Demux/2 -> [acc_mech_trq]

== system lib_accessory/SubLibraries/data logging probes dummy ==
  In1 : Inport
  Terminator : Terminator
  wires:
  In1/1 -> Terminator/1

== system lib_accessory/SubLibraries/data logging probes for conventional mechanical loads ==
  In1 : Inport
  Demux : Demux  Outputs=12
  To Workspace : ToWorkspace  VariableName=acc_ac_pwr_out_a  SampleTime=-1
  To Workspace1 : ToWorkspace  VariableName=acc_pwr_steer_pwr_out_a  SampleTime=-1
  To Workspace10 : ToWorkspace  VariableName=acc_op_pwr_out_a  SampleTime=-1
  To Workspace11 : ToWorkspace  VariableName=acc_op_duty  SampleTime=-1
  To Workspace2 : ToWorkspace  VariableName=acc_air_comp_pwr_out_a  SampleTime=-1
  To Workspace3 : ToWorkspace  VariableName=acc_eng_fan_pwr_out_a  SampleTime=-1
  To Workspace4 : ToWorkspace  VariableName=acc_alt_pwr_out_a  SampleTime=-1
  To Workspace5 : ToWorkspace  VariableName=acc_14elec_pwr_out_a  SampleTime=-1
  To Workspace6 : ToWorkspace  VariableName=acc_ps_duty  SampleTime=-1
  To Workspace7 : ToWorkspace  VariableName=acc_air_comp_duty  SampleTime=-1
  To Workspace8 : ToWorkspace  VariableName=acc_fan_duty  SampleTime=-1
  To Workspace9 : ToWorkspace  VariableName=acc_ac_duty  SampleTime=-1
  wires:
  Demux/12 -> To Workspace11/1
  Demux/11 -> To Workspace10/1
  Demux/10 -> To Workspace9/1
  Demux/9 -> To Workspace8/1
  Demux/8 -> To Workspace7/1
  Demux/7 -> To Workspace6/1
  Demux/6 -> To Workspace5/1
  Demux/5 -> To Workspace4/1
  Demux/4 -> To Workspace3/1
  Demux/3 -> To Workspace2/1
  Demux/2 -> To Workspace1/1
  Demux/1 -> To Workspace/1
  In1/1 -> Demux/1

== system lib_accessory/SubLibraries/data probes ==
  In1 : Inport
  data logging probes for conventional mechanical loads : lib_accessory/SubLibraries/data logging probes for conventional mechanical loads
      settings: RTWFcnNameOpts=Auto  RTWFileNameOpts=Auto
  wires:
  In1/1 -> data logging probes for conventional mechanical loads/1

== system lib_accessory/SubLibraries/electrical power logging ==
  In1 : Inport
  Gain : Gain  Gain=acc_elec_eff  SaturateOnIntegerOverflow=on  OutDataTypeStr=Inherit: Same as input  ParamDataTypeStr=Inherit: Same as input
  To Workspace6 : ToWorkspace  VariableName=acc_elec_pwr_in_a  SampleTime=-1
  To Workspace8 : ToWorkspace  VariableName=acc_elec_pwr_out_a  SampleTime=-1
  wires:
  In1/1 -> To Workspace6/1, Gain/1
  Gain/1 -> To Workspace8/1

== system lib_accessory/SubLibraries/mechanical power logging ==
  In1 : Inport
  Gain : Gain  Gain=acc_mech_eff  SaturateOnIntegerOverflow=on  OutDataTypeStr=Inherit: Same as input  ParamDataTypeStr=Inherit: Same as input
  To Workspace6 : ToWorkspace  VariableName=acc_mech_pwr_in_a  SampleTime=-1
  To Workspace8 : ToWorkspace  VariableName=acc_mech_pwr_out_a  SampleTime=-1
  wires:
  In1/1 -> To Workspace6/1, Gain/1
  Gain/1 -> To Workspace8/1

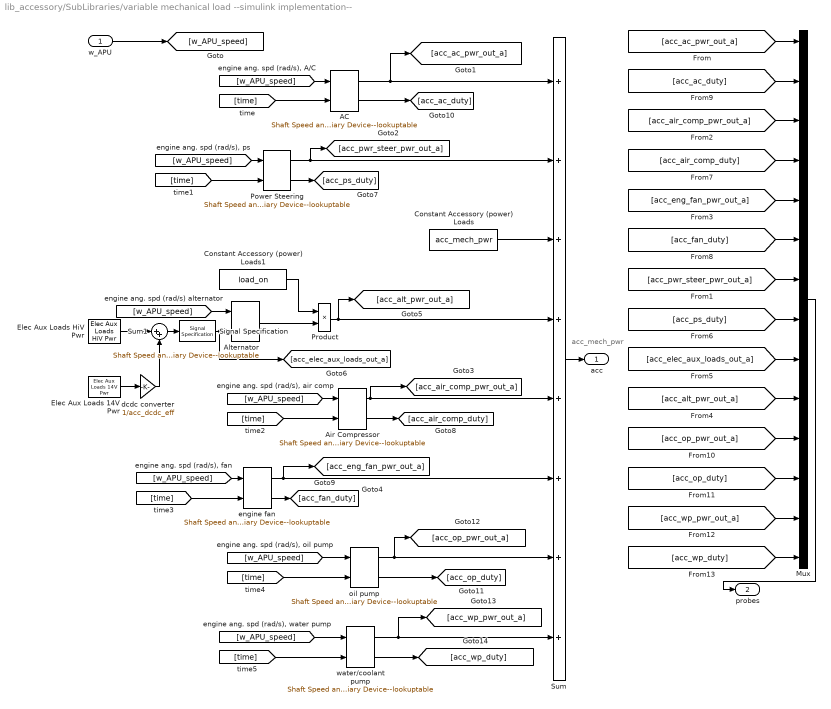
== system lib_accessory/SubLibraries/variable mechanical load --simulink implementation-- ==
  note: acc_mech_pwr
  w_APU : Inport
  AC : lib_accessory/SubLibraries/Shaft Speed and Time Loaded Auxiliary Device--lookuptable  fname=acc_ac_init  acc_duty=acc_ac_dutycycle
  Air Compressor : lib_accessory/SubLibraries/Shaft Speed and Time Loaded Auxiliary Device--lookuptable  fname=acc_abc_init  acc_duty=acc_abc_dutycycle
  Alternator : lib_accessory/SubLibraries/Shaft Speed and Actual Load Auxiliary Device--lookuptable  conv_eff=acc_acdc_inverter_eff  fname=acc_alt_init
  Constant Accessory (power) Loads : Constant  Value=acc_mech_pwr
  Constant Accessory (power) Loads1 : Constant  Value=load_on
  Elec Aux Loads 14V Pwr : lib_accessory/Elec Aux Loads 14V Pwr
  Elec Aux Loads HiV Pwr : lib_accessory/Elec Aux Loads HiV Pwr
  Mux : Mux  Inputs=14
  Power Steering : lib_accessory/SubLibraries/Shaft Speed and Time Loaded Auxiliary Device--lookuptable  fname=acc_ps_init  acc_duty=acc_ps_dutycycle
  Product : Product  SaturateOnIntegerOverflow=on  RndMeth=Zero  InputSameDT=on  OutDataTypeStr=Inherit: Same as first input
  Signal Specification : SignalSpecification  Dimensions=1
  Sum : Sum  Inputs=++++++++  SaturateOnIntegerOverflow=on  InputSameDT=on  OutDataTypeStr=Inherit: Same as first input
  Sum1 : Sum  Inputs=|++  SaturateOnIntegerOverflow=on  InputSameDT=on  OutDataTypeStr=Inherit: Same as first input
  dcdc converter : Gain  Gain=1/acc_dcdc_eff  SaturateOnIntegerOverflow=on  OutDataTypeStr=Inherit: Same as input  ParamDataTypeStr=Inherit: Same as input
  engine fan : lib_accessory/SubLibraries/Shaft Speed and Time Loaded Auxiliary Device--lookuptable  fname=acc_ef_init  acc_duty=acc_ef_dutycycle
  oil pump : lib_accessory/SubLibraries/Shaft Speed and Time Loaded Auxiliary Device--lookuptable  fname=acc_op_init  acc_duty=acc_op_dutycycle
  water/coolant pump : lib_accessory/SubLibraries/Shaft Speed and Time Loaded Auxiliary Device--lookuptable  fname=acc_wp_init  acc_duty=acc_wp_dutycycle
  acc : Outport
  probes : Outport  Port=2
  wires:
  [time] -> AC/2
  [w_APU_speed] -> AC/1
  AC/2 -> [acc_ac_duty]
  AC/1 -> Sum/1, [acc_ac_pwr_out_a]
  Constant Accessory (power) Loads/1 -> Sum/3
  Sum/1 -> acc/1
  [w_APU_speed] -> Alternator/1
  Air Compressor/2 -> [acc_air_comp_duty]
  Air Compressor/1 -> Sum/5, [acc_air_comp_pwr_out_a]
  [w_APU_speed] -> Air Compressor/1
  [time] -> Air Compressor/2
  oil pump/1 -> [acc_op_pwr_out_a], Sum/7
  oil pump/2 -> [acc_op_duty]
  [time] -> oil pump/2
  [w_APU_speed] -> oil pump/1
  engine fan/2 -> [acc_fan_duty]
  [time] -> engine fan/2
  engine fan/1 -> Sum/6, [acc_eng_fan_pwr_out_a]
  [w_APU_speed] -> engine fan/1
  Power Steering/2 -> [acc_ps_duty]
  [w_APU_speed] -> Power Steering/1
  [time] -> Power Steering/2
  Power Steering/1 -> Sum/2, [acc_pwr_steer_pwr_out_a]
  w_APU/1 -> [w_APU_speed]
  Elec Aux Loads 14V Pwr/1 -> dcdc converter/1
  Signal Specification/1 -> Alternator/2, [acc_elec_aux_loads_out_a]
  [acc_ac_pwr_out_a] -> Mux/1
  Product/1 -> Sum/4, [acc_alt_pwr_out_a]
  Constant Accessory (power) Loads1/1 -> Product/1
  Alternator/1 -> Product/2
  Mux/1 -> probes/1
  water/coolant pump/1 -> Sum/8, [acc_wp_pwr_out_a]
  [time] -> water/coolant pump/2
  [w_APU_speed] -> water/coolant pump/1
  water/coolant pump/2 -> [acc_wp_duty]
  [acc_ac_duty] -> Mux/2
  [acc_air_comp_pwr_out_a] -> Mux/3
  [acc_air_comp_duty] -> Mux/4
  [acc_eng_fan_pwr_out_a] -> Mux/5
  [acc_fan_duty] -> Mux/6
  [acc_pwr_steer_pwr_out_a] -> Mux/7
  [acc_ps_duty] -> Mux/8
  [acc_elec_aux_loads_out_a] -> Mux/9
  [acc_alt_pwr_out_a] -> Mux/10
  [acc_op_pwr_out_a] -> Mux/11
  [acc_op_duty] -> Mux/12
  [acc_wp_pwr_out_a] -> Mux/13
  [acc_wp_duty] -> Mux/14
  Sum1/1 -> Signal Specification/1
  Elec Aux Loads HiV Pwr/1 -> Sum1/1
  dcdc converter/1 -> Sum1/2

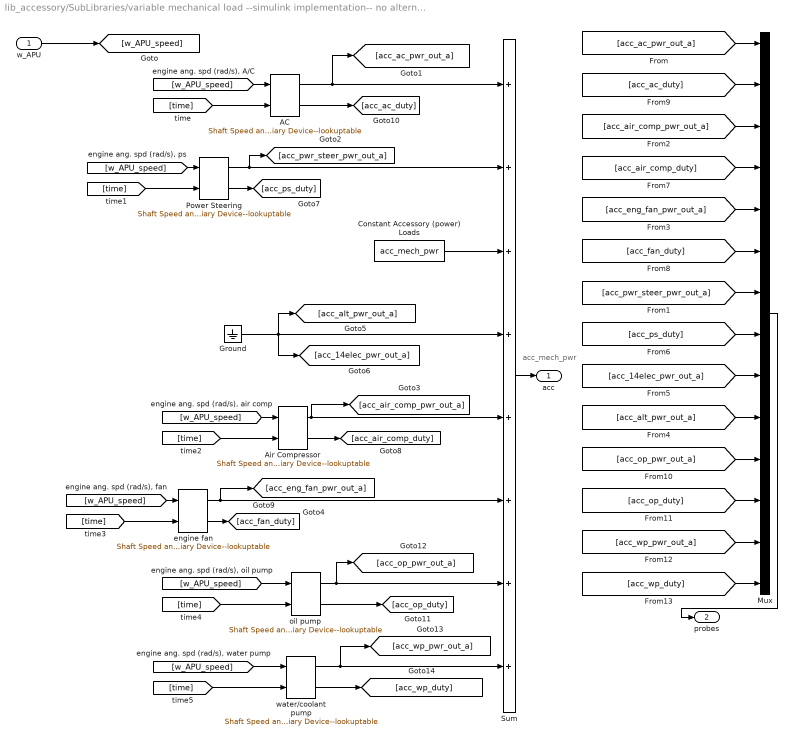
== system lib_accessory/SubLibraries/variable mechanical load --simulink implementation-- no alternator ==
  note: acc_mech_pwr
  w_APU : Inport
  AC : lib_accessory/SubLibraries/Shaft Speed and Time Loaded Auxiliary Device--lookuptable  fname=acc_ac_init  acc_duty=acc_ac_dutycycle
  Air Compressor : lib_accessory/SubLibraries/Shaft Speed and Time Loaded Auxiliary Device--lookuptable  fname=acc_abc_init  acc_duty=acc_abc_dutycycle
  Constant Accessory (power) Loads : Constant  Value=acc_mech_pwr
  Ground : Ground
  Mux : Mux  Inputs=14
  Power Steering : lib_accessory/SubLibraries/Shaft Speed and Time Loaded Auxiliary Device--lookuptable  fname=acc_ps_init  acc_duty=acc_ps_dutycycle
  Sum : Sum  Inputs=++++++++  SaturateOnIntegerOverflow=on  InputSameDT=on  OutDataTypeStr=Inherit: Same as first input
  engine fan : lib_accessory/SubLibraries/Shaft Speed and Time Loaded Auxiliary Device--lookuptable  fname=acc_ef_init  acc_duty=acc_ef_dutycycle
  oil pump : lib_accessory/SubLibraries/Shaft Speed and Time Loaded Auxiliary Device--lookuptable  fname=acc_op_init  acc_duty=acc_op_dutycycle
  water/coolant pump : lib_accessory/SubLibraries/Shaft Speed and Time Loaded Auxiliary Device--lookuptable  fname=acc_wp_init  acc_duty=acc_wp_dutycycle
  acc : Outport
  probes : Outport  Port=2
  wires:
  [time] -> AC/2
  [w_APU_speed] -> AC/1
  AC/2 -> [acc_ac_duty]
  AC/1 -> Sum/1, [acc_ac_pwr_out_a]
  Constant Accessory (power) Loads/1 -> Sum/3
  Sum/1 -> acc/1
  Air Compressor/2 -> [acc_air_comp_duty]
  Air Compressor/1 -> Sum/5, [acc_air_comp_pwr_out_a]
  [w_APU_speed] -> Air Compressor/1
  [time] -> Air Compressor/2
  oil pump/1 -> [acc_op_pwr_out_a], Sum/7
  oil pump/2 -> [acc_op_duty]
  [time] -> oil pump/2
  [w_APU_speed] -> oil pump/1
  engine fan/2 -> [acc_fan_duty]
  [time] -> engine fan/2
  engine fan/1 -> Sum/6, [acc_eng_fan_pwr_out_a]
  [w_APU_speed] -> engine fan/1
  Power Steering/2 -> [acc_ps_duty]
  [w_APU_speed] -> Power Steering/1
  [time] -> Power Steering/2
  Power Steering/1 -> Sum/2, [acc_pwr_steer_pwr_out_a]
  w_APU/1 -> [w_APU_speed]
  [acc_ac_pwr_out_a] -> Mux/1
  Ground/1 -> Sum/4, [acc_alt_pwr_out_a], [acc_14elec_pwr_out_a]
  Mux/1 -> probes/1
  water/coolant pump/1 -> Sum/8, [acc_wp_pwr_out_a]
  [time] -> water/coolant pump/2
  [w_APU_speed] -> water/coolant pump/1
  water/coolant pump/2 -> [acc_wp_duty]
  [acc_ac_duty] -> Mux/2
  [acc_air_comp_pwr_out_a] -> Mux/3
  [acc_air_comp_duty] -> Mux/4
  [acc_eng_fan_pwr_out_a] -> Mux/5
  [acc_fan_duty] -> Mux/6
  [acc_pwr_steer_pwr_out_a] -> Mux/7
  [acc_ps_duty] -> Mux/8
  [acc_14elec_pwr_out_a] -> Mux/9
  [acc_alt_pwr_out_a] -> Mux/10
  [acc_op_pwr_out_a] -> Mux/11
  [acc_op_duty] -> Mux/12
  [acc_wp_pwr_out_a] -> Mux/13
  [acc_wp_duty] -> Mux/14
